simulink model "arxeio2teleia6"  (R2021a)
settings: Solver=ode23tb  StartTime=0.0  StopTime=30  MaxStep=1e-5  RelTol=1e-3
libraries: spsCurrentMeasurementLib x10, spsVoltageMeasurementLib x10, spsSeriesRLCBranchLib x10, spsRMSLib x8, spsControlledVoltageSourceLib x6, spsNeutralLib x5, spsMeanLib x4, simulink x3, spsAsynchronousMachineSIUnitsLib x3, spsACVoltageSourceLib x3, spsGroundLib x2, spsPower3phInstantaneousLib x2
settings Model: Creator=User  LastModifiedBy=epape
settings SolverCC: AlgebraicLoopSolver=TrustRegion
settings DebuggingCC: SFMachineParentedDataDiag=warning  ArithmeticOperatorsInVariantConditions=warning
settings SFSimCC: CustomCodeUndefinedFunction=UseInterfaceOnly

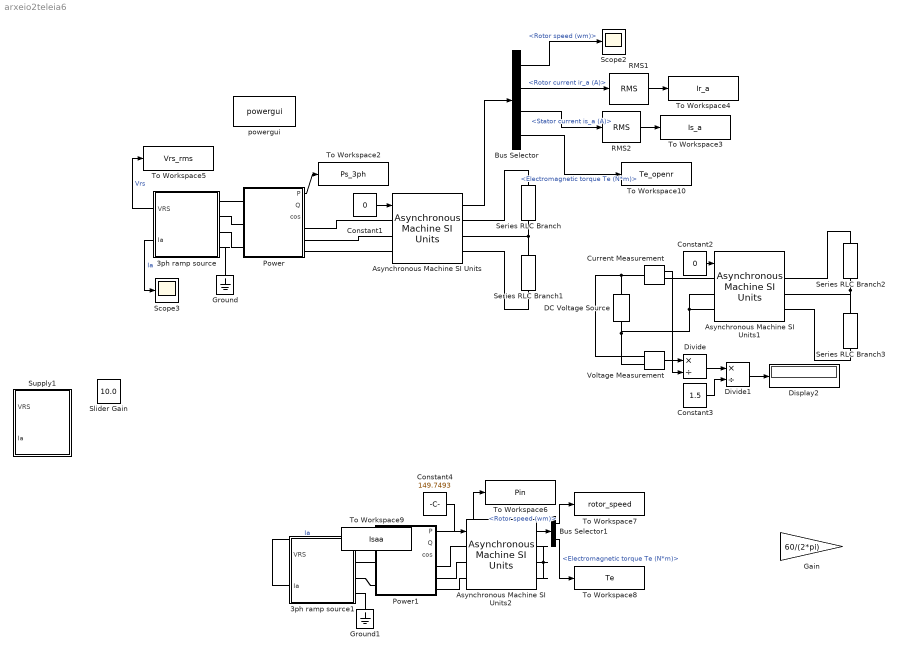
== system arxeio2teleia6 ==
  3ph ramp source : Subsystem  mask{Vrms=400}
      mask prompts: Vrms "LIne Voltage (V)"
  3ph ramp source1 : Subsystem  mask{Vrms=400}
      mask prompts: Vrms "LIne Voltage (V)"
  Asynchronous Machine SI Units : spsAsynchronousMachineSIUnitsLib/Asynchronous Machine SI Units  RotorType=Wound  PresetModel="15:  5.4 HP (4KW)   400 V  50Hz 1430 RPM"  MechanicalLoad=Speed w  ShowDetailedParameters=on  ReferenceFrame=Stationary  Units=SI  MeasurementBus=off  NominalParameters=[4000 400 50]  VoltageRatio=1  Stator=[1.405 0.005839]  Rotor=[1.395 0.005839]  Cage1=[0.4155 0.002066]  Cage2=[0.4168 0.0003495]  Lm=0.1722  Mechanical=[0.0131 0.002985 2]  PolePairs=2  InitialConditions=[1 0 0 0 0 0 0 0]  SimulateSaturation=off  Saturation=[14.03593122, 27.81365428, 53.79336849, 72.68890987, 97.98006896, 148.6815601, 215.7428561, 302.9841135, 428.7778367 ; 230, 322, 414, 460, 506, 552, 598, 644, 690]  LoadFlowParameters=1492000  TsPowergui=0  TsBlock=-1  IterativeModel=Trapezoidal non iterative  IterativeDiscreteModel=Trapezoidal non iterative  Pmec=1.492e+006
  Asynchronous Machine SI Units1 : spsAsynchronousMachineSIUnitsLib/Asynchronous Machine SI Units  RotorType=Wound  PresetModel="15:  5.4 HP (4KW)   400 V  50Hz 1430 RPM"  MechanicalLoad=Speed w  ShowDetailedParameters=on  ReferenceFrame=Stationary  Units=SI  MeasurementBus=off  NominalParameters=[4000 400 50]  VoltageRatio=1  Stator=[1.405 0.005839]  Rotor=[1.395 0.005839]  Cage1=[0.4155 0.002066]  Cage2=[0.4168 0.0003495]  Lm=0.1722  Mechanical=[0.0131 0.002985 2]  PolePairs=2  InitialConditions=[1 0 0 0 0 0 0 0]  SimulateSaturation=off  Saturation=[14.03593122, 27.81365428, 53.79336849, 72.68890987, 97.98006896, 148.6815601, 215.7428561, 302.9841135, 428.7778367 ; 230, 322, 414, 460, 506, 552, 598, 644, 690]  LoadFlowParameters=1492000  TsPowergui=0  TsBlock=-1  IterativeModel=Trapezoidal non iterative  IterativeDiscreteModel=Trapezoidal non iterative  Pmec=1.492e+006
  Asynchronous Machine SI Units2 : spsAsynchronousMachineSIUnitsLib/Asynchronous Machine SI Units  RotorType=Wound  PresetModel="15:  5.4 HP (4KW)   400 V  50Hz 1430 RPM"  MechanicalLoad=Speed w  ShowDetailedParameters=on  ReferenceFrame=Stationary  Units=SI  MeasurementBus=off  NominalParameters=[4000 400 50]  VoltageRatio=1  Stator=[1.405 0.005839]  Rotor=[1.395 0.005839]  Cage1=[0.4155 0.002066]  Cage2=[0.4168 0.0003495]  Lm=0.1722  Mechanical=[0.0131 0.002985 2]  PolePairs=2  InitialConditions=[1 0 0 0 0 0 0 0]  SimulateSaturation=off  Saturation=[14.03593122, 27.81365428, 53.79336849, 72.68890987, 97.98006896, 148.6815601, 215.7428561, 302.9841135, 428.7778367 ; 230, 322, 414, 460, 506, 552, 598, 644, 690]  LoadFlowParameters=1492000  TsPowergui=0  TsBlock=-1  IterativeModel=Trapezoidal non iterative  IterativeDiscreteModel=Trapezoidal non iterative  Pmec=1.492e+006
  Bus Selector : BusSelector  OutputSignals=Mechanical.Rotor speed (wm),Rotor measurements.Rotor current ir_a (A),Stator measurements.Stator current is_a (A),Mechanical.Electromagnetic torque Te (N*m)
  Bus Selector1 : BusSelector  OutputSignals=Mechanical.Rotor speed (wm),Mechanical.Electromagnetic torque Te (N*m)
  Constant1 : Constant  Value=0
  Constant2 : Constant  Value=0
  Constant3 : Constant  Value=1.5
  Constant4 : Constant  Value=149.7493
  Current Measurement : spsCurrentMeasurementLib/Current Measurement  PhasorSimulation=off  OutputType=Complex  PSBequivalent=0
  DC Voltage Source : spsDCVoltageSourceLib/DC Voltage Source  Amplitude=16.2235  Measurements=None
  Display2 : Display
  Divide : Product  Inputs=*/
  Divide1 : Product  Inputs=*/
  Gain : Gain  Gain=60/(2*pi)
  Ground : spsGroundLib/Ground  LConnTagsString=a
  Ground1 : spsGroundLib/Ground  LConnTagsString=a
  Power : Subsystem
      mask DialogControl Control2 Prompt: Three phase power measurement
  Power1 : Subsystem
      mask DialogControl Control2 Prompt: Three phase power measurement
  RMS1 : spsRMSLib/RMS  TrueRMS=on  Freq=50  RMSInit=0  Ts=0
  RMS2 : spsRMSLib/RMS  TrueRMS=on  Freq=50  RMSInit=0  Ts=0
  Scope2 : Scope
  Scope3 : Scope
  Series RLC Branch{,1..3} (4 alike) : spsSeriesRLCBranchLib/Series RLC Branch  LConnTagsString=__new0  RConnTagsString=__new0  BranchType=R  Resistance=1e6  Inductance=1e-3  SetiL0=off  InitialCurrent=0  Capacitance=1e-6  Setx0=off  InitialVoltage=0  Measurements=None
  Slider Gain : simulink/Math Operations/Slider Gain  gain=10.0  low=0  high=10
  Supply1 : Subsystem  mask{VLL=400}
      mask prompts: VLL "Line Voltage (V)"
      mask DialogControl Label1 Prompt: 3 phase power supply
  To Workspace10 : ToWorkspace  VariableName=Te_openr  SaveFormat=Timeseries  SampleTime=-1
  To Workspace2 : ToWorkspace  VariableName=Ps_3ph  SaveFormat=Timeseries  SampleTime=-1
  To Workspace3 : ToWorkspace  VariableName=Is_a  SaveFormat=Timeseries  SampleTime=-1
  To Workspace4 : ToWorkspace  VariableName=Ir_a  SaveFormat=Timeseries  SampleTime=-1
  To Workspace5 : ToWorkspace  VariableName=Vrs_rms  SaveFormat=Timeseries  SampleTime=-1
  To Workspace6 : ToWorkspace  VariableName=Pin  SaveFormat=Timeseries  SampleTime=-1
  To Workspace7 : ToWorkspace  VariableName=rotor_speed  SaveFormat=Timeseries  SampleTime=-1
  To Workspace8 : ToWorkspace  VariableName=Te  SaveFormat=Timeseries  SampleTime=-1
  To Workspace9 : ToWorkspace  VariableName=Isaa  SaveFormat=Timeseries  SampleTime=-1
  Voltage Measurement : spsVoltageMeasurementLib/Voltage Measurement  PhasorSimulation=off  OutputType=Complex  PSBequivalent=0
  powergui : spspowerguiLib/powergui  Priority=1  SimulationMode=Continuous  SampleTime=50e-6  frequency=60  Iterations=50  frequencyindice=50  Pbase=100e6  ErrMax=1e-4  UnitsV=kV  UnitsW=MW  buscounter=0  FunctionMessages=off  echomessages=off  EnableUseOfTLC=off  CurrentSourceSwitches=off  DisableSnubberDevices=off  DisableRonSwitches=off  DisableVfSwitches=off  DisplayEquations=off  AutomaticDiscreteSolvers=off  SolverType=Tustin/Backward Euler (TBE)  Interpol=off  ExternalGateDelay=off  methode=off  Ts=100  x0status=blocks  SPID=on  SwTol=0  HookPort=off  NonlinearTolerance=1e-4  nMaxIteration=100  ContinueOnMaxIteration=off  RestoreLinks=warning  ResistiveCurrentMeasurement=off  Frange=[0:2:500]  Ylog=off  Xlog=on  ShowGrid=off  save=off  variable=ZData  structure=0  ZoomFFT=off  StartTime=0.0  cycles=1  DisplayStyle=1  fundamental=60  FreqAxis=off  MaxFrequency=1000  frequencyindicesteady=1  RmsSteady=1  display=off
  wires:
  Asynchronous Machine SI Units/1 -> Bus Selector/1
  Bus Selector/3 -> RMS2/1  "<Stator current is_a (A)>"
  Bus Selector/2 -> RMS1/1  "<Rotor current ir_a (A)>"
  RMS2/1 -> To Workspace3/1
  RMS1/1 -> To Workspace4/1
  Bus Selector/1 -> Scope2/1  "<Rotor speed (wm)>"
  Constant1/1 -> Asynchronous Machine SI Units/1
  3ph ramp source/2(Ia) -> Scope3/1  "Ia"
  Power/1(P) -> To Workspace2/1
  3ph ramp source/1(VRS) -> To Workspace5/1  "Vrs"
  Bus Selector/4 -> To Workspace10/1  "<Electromagnetic torque Te (N*m)>"
  Power1/1(P) -> To Workspace6/1
  Bus Selector1/1 -> To Workspace7/1  "<Rotor speed (wm)>"
  Constant3/1 -> Divide1/2
  Voltage Measurement/1 -> Divide/1
  Constant4/1 -> Asynchronous Machine SI Units2/1
  Bus Selector1/2 -> To Workspace8/1  "<Electromagnetic torque Te (N*m)>"
  3ph ramp source1/2(Ia) -> To Workspace9/1  "Ia"
  Asynchronous Machine SI Units2/1 -> Bus Selector1/1
  Divide/1 -> Divide1/1
  Current Measurement/1 -> Divide/2
  Divide1/1 -> Display2/1
  Constant2/1 -> Asynchronous Machine SI Units1/1
  connections:
  Series RLC Branch/LConn1 -- Asynchronous Machine SI Units/RConn1
  Asynchronous Machine SI Units/RConn2 -- Series RLC Branch1/LConn1 -- Series RLC Branch/RConn1
  Series RLC Branch1/RConn1 -- Asynchronous Machine SI Units/RConn3
  Power/LConn2 -- 3ph ramp source/LConn2
  Power/LConn1 -- 3ph ramp source/LConn1
  Power/RConn1 -- Asynchronous Machine SI Units/LConn1
  Power/RConn2 -- Asynchronous Machine SI Units/LConn2
  Power/RConn3 -- Asynchronous Machine SI Units/LConn3
  3ph ramp source/LConn3 -- Power/LConn3
  3ph ramp source/LConn4 -- Ground/LConn1
  Voltage Measurement/LConn2 -- Asynchronous Machine SI Units1/LConn3 -- Asynchronous Machine SI Units1/LConn2 -- DC Voltage Source/LConn1
  Series RLC Branch2/RConn1 -- Series RLC Branch3/LConn1 -- Asynchronous Machine SI Units1/RConn2
  Voltage Measurement/LConn1 -- Current Measurement/LConn1 -- DC Voltage Source/RConn1
  Asynchronous Machine SI Units2/RConn1 -- Asynchronous Machine SI Units2/RConn3 -- Asynchronous Machine SI Units2/RConn2
  3ph ramp source1/LConn2 -- Power1/LConn2
  Power1/RConn1 -- Asynchronous Machine SI Units2/LConn1
  3ph ramp source1/LConn3 -- Power1/LConn3
  Power1/RConn2 -- Asynchronous Machine SI Units2/LConn2
  3ph ramp source1/LConn4 -- Ground1/LConn1
  3ph ramp source1/LConn1 -- Power1/LConn1
  Power1/RConn3 -- Asynchronous Machine SI Units2/LConn3
  Asynchronous Machine SI Units1/RConn3 -- Series RLC Branch3/RConn1
  Series RLC Branch2/LConn1 -- Asynchronous Machine SI Units1/RConn1
  Current Measurement/RConn1 -- Asynchronous Machine SI Units1/LConn1

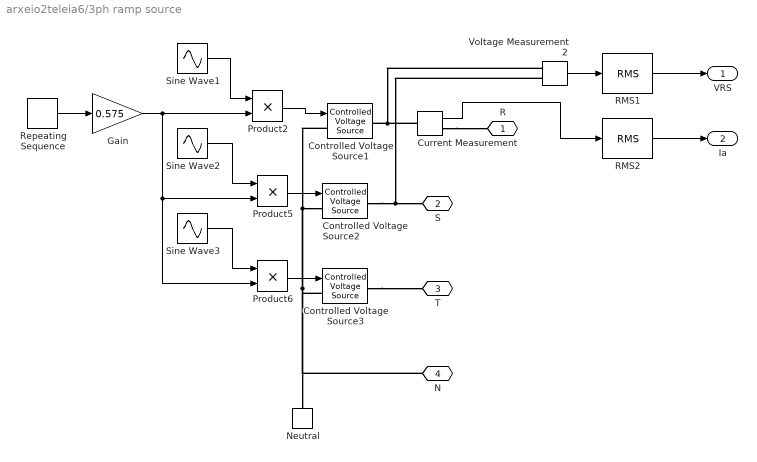
== system arxeio2teleia6/3ph ramp source ==
  Controlled Voltage Source1 : spsControlledVoltageSourceLib/Controlled Voltage Source  Initialize=on  Source_Type=AC  Amplitude=0  Phase=0  Frequency=50  Measurements=Voltage
  Controlled Voltage Source2 : spsControlledVoltageSourceLib/Controlled Voltage Source  Initialize=on  Source_Type=AC  Amplitude=0  Phase=0  Frequency=50  Measurements=Voltage
  Controlled Voltage Source3 : spsControlledVoltageSourceLib/Controlled Voltage Source  Initialize=on  Source_Type=AC  Amplitude=0  Phase=0  Frequency=50  Measurements=Voltage
  Current Measurement : spsCurrentMeasurementLib/Current Measurement  PhasorSimulation=off  OutputType=Complex  PSBequivalent=0
  Gain : Gain  Gain=0.575
  Neutral : spsNeutralLib/Neutral  LConnTagsString=a  NodeNumber=10
      settings: AttributesFormatString=node %<NodeNumber>  SourceProductBaseCode=PS
  Product2 : Product
  Product5 : Product
  Product6 : Product
  RMS1 : spsRMSLib/RMS  TrueRMS=on  Freq=50  RMSInit=0  Ts=0
  RMS2 : spsRMSLib/RMS  TrueRMS=on  Freq=50  RMSInit=0  Ts=0
  Repeating Sequence : simulink/Sources/Repeating Sequence  rep_seq_t=t  rep_seq_y=Vs
  Sine Wave1 : Sin  Amplitude=sqrt(2)  Frequency=100*pi  SampleTime=0
  Sine Wave2 : Sin  Amplitude=sqrt(2)  Frequency=100*pi  Phase=-2*pi/3  SampleTime=0
  Sine Wave3 : Sin  Amplitude=sqrt(2)  Frequency=100*pi  Phase=2*pi/3  SampleTime=0
  Voltage Measurement2 : spsVoltageMeasurementLib/Voltage Measurement  PhasorSimulation=off  OutputType=Complex  PSBequivalent=0
  R : PMIOPort  Side=Left
  S : PMIOPort  Port=2  Side=Left
  T : PMIOPort  Port=3  Side=Left
  N : PMIOPort  Port=4  Side=Left
  VRS : Outport
  Ia : Outport  Port=2
  wires:
  Repeating Sequence/1 -> Gain/1
  Product5/1 -> Controlled Voltage Source2/1
  Sine Wave2/1 -> Product5/1
  Product6/1 -> Controlled Voltage Source3/1
  Sine Wave3/1 -> Product6/1
  Product2/1 -> Controlled Voltage Source1/1
  Sine Wave1/1 -> Product2/1
  Gain/1 -> Product6/2, Product5/2, Product2/2
  Voltage Measurement2/1 -> RMS1/1
  Current Measurement/1 -> RMS2/1
  RMS2/1 -> Ia/1
  RMS1/1 -> VRS/1
  connections:
  Controlled Voltage Source2/RConn1 -- Voltage Measurement2/LConn2 -- S/RConn1
  Controlled Voltage Source1/LConn1 -- Controlled Voltage Source2/LConn1 -- Controlled Voltage Source3/LConn1 -- N/RConn1 -- Neutral/LConn1
  Controlled Voltage Source3/RConn1 -- T/RConn1
  Current Measurement/RConn1 -- R/RConn1
  Current Measurement/LConn1 -- Voltage Measurement2/LConn1 -- Controlled Voltage Source1/RConn1

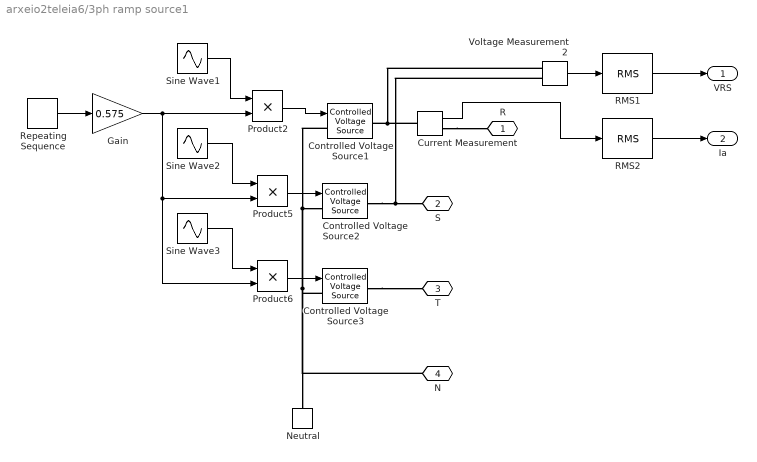
== system arxeio2teleia6/3ph ramp source1 ==
  Controlled Voltage Source1 : spsControlledVoltageSourceLib/Controlled Voltage Source  Initialize=on  Source_Type=AC  Amplitude=0  Phase=0  Frequency=50  Measurements=Voltage
  Controlled Voltage Source2 : spsControlledVoltageSourceLib/Controlled Voltage Source  Initialize=on  Source_Type=AC  Amplitude=0  Phase=0  Frequency=50  Measurements=Voltage
  Controlled Voltage Source3 : spsControlledVoltageSourceLib/Controlled Voltage Source  Initialize=on  Source_Type=AC  Amplitude=0  Phase=0  Frequency=50  Measurements=Voltage
  Current Measurement : spsCurrentMeasurementLib/Current Measurement  PhasorSimulation=off  OutputType=Complex  PSBequivalent=0
  Gain : Gain  Gain=0.575
  Neutral : spsNeutralLib/Neutral  LConnTagsString=a  NodeNumber=10
      settings: AttributesFormatString=node %<NodeNumber>  SourceProductBaseCode=PS
  Product2 : Product
  Product5 : Product
  Product6 : Product
  RMS1 : spsRMSLib/RMS  TrueRMS=on  Freq=50  RMSInit=0  Ts=0
  RMS2 : spsRMSLib/RMS  TrueRMS=on  Freq=50  RMSInit=0  Ts=0
  Repeating Sequence : simulink/Sources/Repeating Sequence  rep_seq_t=[0 5]  rep_seq_y=[400 400]
  Sine Wave1 : Sin  Amplitude=sqrt(2)  Frequency=100*pi  SampleTime=0
  Sine Wave2 : Sin  Amplitude=sqrt(2)  Frequency=100*pi  Phase=-2*pi/3  SampleTime=0
  Sine Wave3 : Sin  Amplitude=sqrt(2)  Frequency=100*pi  Phase=2*pi/3  SampleTime=0
  Voltage Measurement2 : spsVoltageMeasurementLib/Voltage Measurement  PhasorSimulation=off  OutputType=Complex  PSBequivalent=0
  R : PMIOPort  Side=Left
  S : PMIOPort  Port=2  Side=Left
  T : PMIOPort  Port=3  Side=Left
  N : PMIOPort  Port=4  Side=Left
  VRS : Outport
  Ia : Outport  Port=2
  wires:
  Repeating Sequence/1 -> Gain/1
  Product5/1 -> Controlled Voltage Source2/1
  Sine Wave2/1 -> Product5/1
  Product6/1 -> Controlled Voltage Source3/1
  Sine Wave3/1 -> Product6/1
  Product2/1 -> Controlled Voltage Source1/1
  Sine Wave1/1 -> Product2/1
  Gain/1 -> Product6/2, Product5/2, Product2/2
  Voltage Measurement2/1 -> RMS1/1
  Current Measurement/1 -> RMS2/1
  RMS2/1 -> Ia/1
  RMS1/1 -> VRS/1
  connections:
  Controlled Voltage Source2/RConn1 -- Voltage Measurement2/LConn2 -- S/RConn1
  Controlled Voltage Source1/LConn1 -- Controlled Voltage Source2/LConn1 -- Controlled Voltage Source3/LConn1 -- N/RConn1 -- Neutral/LConn1
  Controlled Voltage Source3/RConn1 -- T/RConn1
  Current Measurement/RConn1 -- R/RConn1
  Current Measurement/LConn1 -- Voltage Measurement2/LConn1 -- Controlled Voltage Source1/RConn1

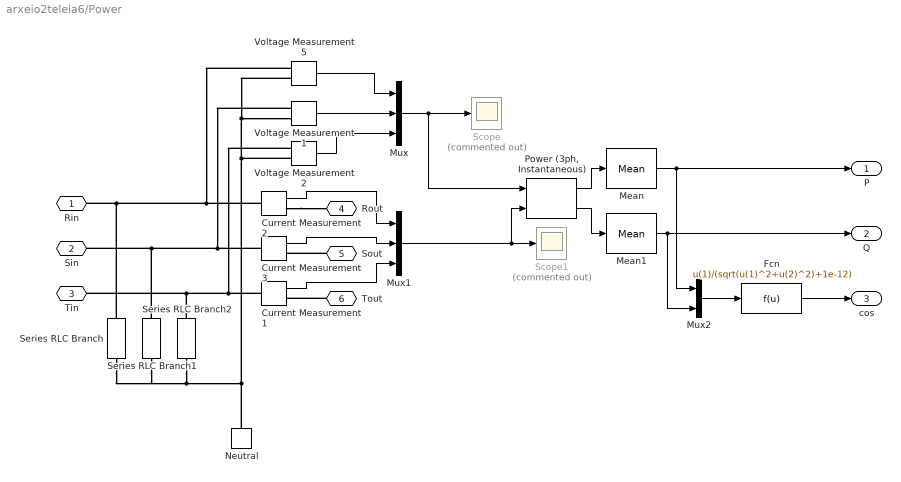
== system arxeio2teleia6/Power ==
  Current Measurement1 : spsCurrentMeasurementLib/Current Measurement  PhasorSimulation=off  OutputType=Complex  PSBequivalent=0
  Current Measurement2 : spsCurrentMeasurementLib/Current Measurement  PhasorSimulation=off  OutputType=Complex  PSBequivalent=0
  Current Measurement3 : spsCurrentMeasurementLib/Current Measurement  PhasorSimulation=off  OutputType=Complex  PSBequivalent=0
  Fcn : Fcn  Expr=u(1)/(sqrt(u(1)^2+u(2)^2)+1e-12)
  Mean : spsMeanLib/Mean  Freq=50  Vinit=0  Ts=0
  Mean1 : spsMeanLib/Mean  Freq=50  Vinit=0  Ts=0
  Mux : Mux  Inputs=3
  Mux1 : Mux  Inputs=3
  Mux2 : Mux  Inputs=2
  Neutral : spsNeutralLib/Neutral  LConnTagsString=a  NodeNumber=10
      settings: AttributesFormatString=node %<NodeNumber>  SourceProductBaseCode=PS
  "Power (3ph, Instantaneous)" : spsPower3phInstantaneousLib/Power (3ph, Instantaneous)
  Scope : Scope  Commented=on
  Scope1 : Scope  Commented=on
  Series RLC Branch : spsSeriesRLCBranchLib/Series RLC Branch  LConnTagsString=__new0  RConnTagsString=__new0  BranchType=R  Resistance=1e6  Inductance=1e-3  SetiL0=off  InitialCurrent=0  Capacitance=1e-6  Setx0=off  InitialVoltage=0  Measurements=None
  Series RLC Branch1 : spsSeriesRLCBranchLib/Series RLC Branch  LConnTagsString=__new0  RConnTagsString=__new0  BranchType=R  Resistance=1e6  Inductance=1e-3  SetiL0=off  InitialCurrent=0  Capacitance=1e-6  Setx0=off  InitialVoltage=0  Measurements=None
  Series RLC Branch2 : spsSeriesRLCBranchLib/Series RLC Branch  LConnTagsString=__new0  RConnTagsString=__new0  BranchType=R  Resistance=1e6  Inductance=1e-3  SetiL0=off  InitialCurrent=0  Capacitance=1e-6  Setx0=off  InitialVoltage=0  Measurements=None
  Voltage Measurement1 : spsVoltageMeasurementLib/Voltage Measurement  PhasorSimulation=off  OutputType=Complex  PSBequivalent=0
  Voltage Measurement2 : spsVoltageMeasurementLib/Voltage Measurement  PhasorSimulation=off  OutputType=Complex  PSBequivalent=0
  Voltage Measurement5 : spsVoltageMeasurementLib/Voltage Measurement  PhasorSimulation=off  OutputType=Complex  PSBequivalent=0
  Rin : PMIOPort  Side=Left
  Sin : PMIOPort  Port=2  Side=Left
  Tin : PMIOPort  Port=3  Side=Left
  Rout : PMIOPort  Port=4  Side=Right
  Sout : PMIOPort  Port=5  Side=Right
  Tout : PMIOPort  Port=6  Side=Right
  P : Outport
  Q : Outport  Port=2
  cos : Outport  Port=3
  wires:
  "Power (3ph, Instantaneous)"/1 -> Mean/1
  Mux/1 -> "Power (3ph, Instantaneous)"/1, Scope/1
  Voltage Measurement5/1 -> Mux/1
  Voltage Measurement1/1 -> Mux/2
  Voltage Measurement2/1 -> Mux/3
  Current Measurement3/1 -> Mux1/2
  Current Measurement2/1 -> Mux1/1
  Current Measurement1/1 -> Mux1/3
  "Power (3ph, Instantaneous)"/2 -> Mean1/1
  Mean/1 -> Mux2/1, P/1
  Mux2/1 -> Fcn/1
  Fcn/1 -> cos/1
  Mean1/1 -> Mux2/2, Q/1
  Mux1/1 -> "Power (3ph, Instantaneous)"/2, Scope1/1
  connections:
  Current Measurement1/LConn1 -- Voltage Measurement2/LConn1 -- Series RLC Branch2/LConn1 -- Tin/RConn1
  Current Measurement3/LConn1 -- Voltage Measurement1/LConn1 -- Series RLC Branch1/LConn1 -- Sin/RConn1
  Current Measurement2/LConn1 -- Voltage Measurement5/LConn1 -- Series RLC Branch/LConn1 -- Rin/RConn1
  Voltage Measurement5/LConn2 -- Series RLC Branch/RConn1 -- Series RLC Branch1/RConn1 -- Series RLC Branch2/RConn1 -- Neutral/LConn1 -- Voltage Measurement2/LConn2 -- Voltage Measurement1/LConn2
  Current Measurement2/RConn1 -- Rout/RConn1
  Sout/RConn1 -- Current Measurement3/RConn1
  Tout/RConn1 -- Current Measurement1/RConn1

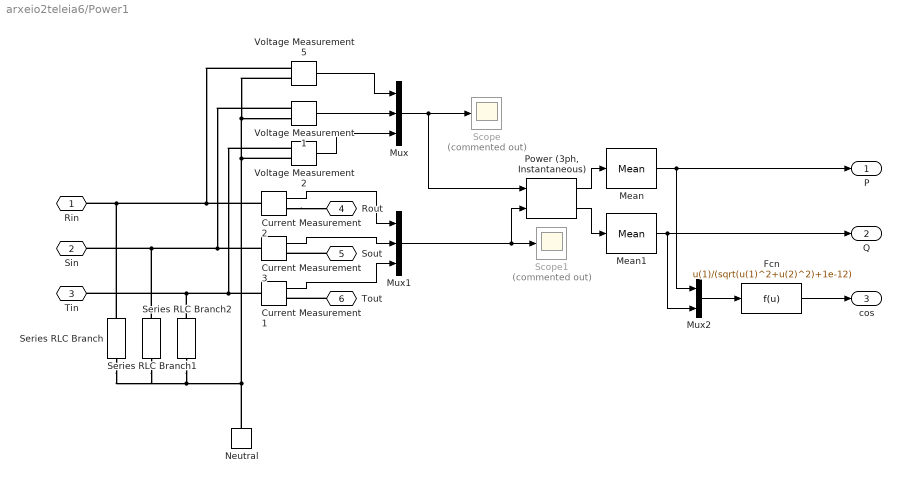
== system arxeio2teleia6/Power1 ==
  Current Measurement1 : spsCurrentMeasurementLib/Current Measurement  PhasorSimulation=off  OutputType=Complex  PSBequivalent=0
  Current Measurement2 : spsCurrentMeasurementLib/Current Measurement  PhasorSimulation=off  OutputType=Complex  PSBequivalent=0
  Current Measurement3 : spsCurrentMeasurementLib/Current Measurement  PhasorSimulation=off  OutputType=Complex  PSBequivalent=0
  Fcn : Fcn  Expr=u(1)/(sqrt(u(1)^2+u(2)^2)+1e-12)
  Mean : spsMeanLib/Mean  Freq=50  Vinit=0  Ts=0
  Mean1 : spsMeanLib/Mean  Freq=50  Vinit=0  Ts=0
  Mux : Mux  Inputs=3
  Mux1 : Mux  Inputs=3
  Mux2 : Mux  Inputs=2
  Neutral : spsNeutralLib/Neutral  LConnTagsString=a  NodeNumber=10
      settings: AttributesFormatString=node %<NodeNumber>  SourceProductBaseCode=PS
  "Power (3ph, Instantaneous)" : spsPower3phInstantaneousLib/Power (3ph, Instantaneous)
  Scope : Scope  Commented=on
  Scope1 : Scope  Commented=on
  Series RLC Branch : spsSeriesRLCBranchLib/Series RLC Branch  LConnTagsString=__new0  RConnTagsString=__new0  BranchType=R  Resistance=1e6  Inductance=1e-3  SetiL0=off  InitialCurrent=0  Capacitance=1e-6  Setx0=off  InitialVoltage=0  Measurements=None
  Series RLC Branch1 : spsSeriesRLCBranchLib/Series RLC Branch  LConnTagsString=__new0  RConnTagsString=__new0  BranchType=R  Resistance=1e6  Inductance=1e-3  SetiL0=off  InitialCurrent=0  Capacitance=1e-6  Setx0=off  InitialVoltage=0  Measurements=None
  Series RLC Branch2 : spsSeriesRLCBranchLib/Series RLC Branch  LConnTagsString=__new0  RConnTagsString=__new0  BranchType=R  Resistance=1e6  Inductance=1e-3  SetiL0=off  InitialCurrent=0  Capacitance=1e-6  Setx0=off  InitialVoltage=0  Measurements=None
  Voltage Measurement1 : spsVoltageMeasurementLib/Voltage Measurement  PhasorSimulation=off  OutputType=Complex  PSBequivalent=0
  Voltage Measurement2 : spsVoltageMeasurementLib/Voltage Measurement  PhasorSimulation=off  OutputType=Complex  PSBequivalent=0
  Voltage Measurement5 : spsVoltageMeasurementLib/Voltage Measurement  PhasorSimulation=off  OutputType=Complex  PSBequivalent=0
  Rin : PMIOPort  Side=Left
  Sin : PMIOPort  Port=2  Side=Left
  Tin : PMIOPort  Port=3  Side=Left
  Rout : PMIOPort  Port=4  Side=Right
  Sout : PMIOPort  Port=5  Side=Right
  Tout : PMIOPort  Port=6  Side=Right
  P : Outport
  Q : Outport  Port=2
  cos : Outport  Port=3
  wires:
  "Power (3ph, Instantaneous)"/1 -> Mean/1
  Mux/1 -> "Power (3ph, Instantaneous)"/1, Scope/1
  Voltage Measurement5/1 -> Mux/1
  Voltage Measurement1/1 -> Mux/2
  Voltage Measurement2/1 -> Mux/3
  Current Measurement3/1 -> Mux1/2
  Current Measurement2/1 -> Mux1/1
  Current Measurement1/1 -> Mux1/3
  "Power (3ph, Instantaneous)"/2 -> Mean1/1
  Mean/1 -> Mux2/1, P/1
  Mux2/1 -> Fcn/1
  Fcn/1 -> cos/1
  Mean1/1 -> Mux2/2, Q/1
  Mux1/1 -> "Power (3ph, Instantaneous)"/2, Scope1/1
  connections:
  Current Measurement1/LConn1 -- Voltage Measurement2/LConn1 -- Series RLC Branch2/LConn1 -- Tin/RConn1
  Current Measurement3/LConn1 -- Voltage Measurement1/LConn1 -- Series RLC Branch1/LConn1 -- Sin/RConn1
  Current Measurement2/LConn1 -- Voltage Measurement5/LConn1 -- Series RLC Branch/LConn1 -- Rin/RConn1
  Voltage Measurement5/LConn2 -- Series RLC Branch/RConn1 -- Series RLC Branch1/RConn1 -- Series RLC Branch2/RConn1 -- Neutral/LConn1 -- Voltage Measurement2/LConn2 -- Voltage Measurement1/LConn2
  Current Measurement2/RConn1 -- Rout/RConn1
  Sout/RConn1 -- Current Measurement3/RConn1
  Tout/RConn1 -- Current Measurement1/RConn1

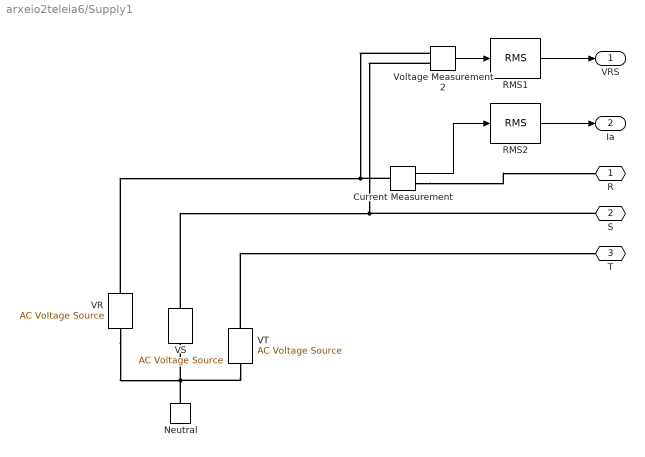
== system arxeio2teleia6/Supply1 ==
  Current Measurement : spsCurrentMeasurementLib/Current Measurement  PhasorSimulation=off  OutputType=Complex  PSBequivalent=0
  Neutral : spsNeutralLib/Neutral  LConnTagsString=a  NodeNumber=10
      settings: AttributesFormatString=node %<NodeNumber>  SourceProductBaseCode=PS
  RMS1 : spsRMSLib/RMS  TrueRMS=on  Freq=50  RMSInit=0  Ts=0
  RMS2 : spsRMSLib/RMS  TrueRMS=on  Freq=50  RMSInit=0  Ts=0
  VR : spsACVoltageSourceLib/AC Voltage Source  Amplitude=VLL*sqrt(2/3)  Phase=0  Frequency=50  SampleTime=0  Measurements=None  BusType=swing  Pref=10e3  Qref=0  Qmin=-inf  Qmax=+inf
  VS : spsACVoltageSourceLib/AC Voltage Source  Amplitude=VLL*sqrt(2/3)  Phase=-120  Frequency=50  SampleTime=0  Measurements=None  BusType=swing  Pref=10e3  Qref=0  Qmin=-inf  Qmax=+inf
  VT : spsACVoltageSourceLib/AC Voltage Source  Amplitude=VLL*sqrt(2/3)  Phase=120  Frequency=50  SampleTime=0  Measurements=None  BusType=swing  Pref=10e3  Qref=0  Qmin=-inf  Qmax=+inf
  Voltage Measurement2 : spsVoltageMeasurementLib/Voltage Measurement  PhasorSimulation=off  OutputType=Complex  PSBequivalent=0
  R : PMIOPort  Side=Left
  S : PMIOPort  Port=2  Side=Left
  T : PMIOPort  Port=3  Side=Left
  VRS : Outport
  Ia : Outport  Port=2
  wires:
  RMS2/1 -> Ia/1
  Current Measurement/1 -> RMS2/1
  RMS1/1 -> VRS/1
  Voltage Measurement2/1 -> RMS1/1
  connections:
  Neutral/LConn1 -- VS/LConn1 -- VT/LConn1 -- VR/LConn1
  S/RConn1 -- VS/RConn1 -- Voltage Measurement2/LConn2
  VT/RConn1 -- T/RConn1
  Current Measurement/LConn1 -- VR/RConn1 -- Voltage Measurement2/LConn1
  Current Measurement/RConn1 -- R/RConn1
